simulink model "vaja04"  (R2013a)
settings: Solver=ode45  StartTime=0.0  StopTime=400  MaxStep=0.01  RelTol=1e-3
undefined symbols (not defined in the file or in its folder): bar, histogram_hitrost, norma
libraries: simulink x39
settings Model: Creator=Studenti  LastModifiedBy=Studenti

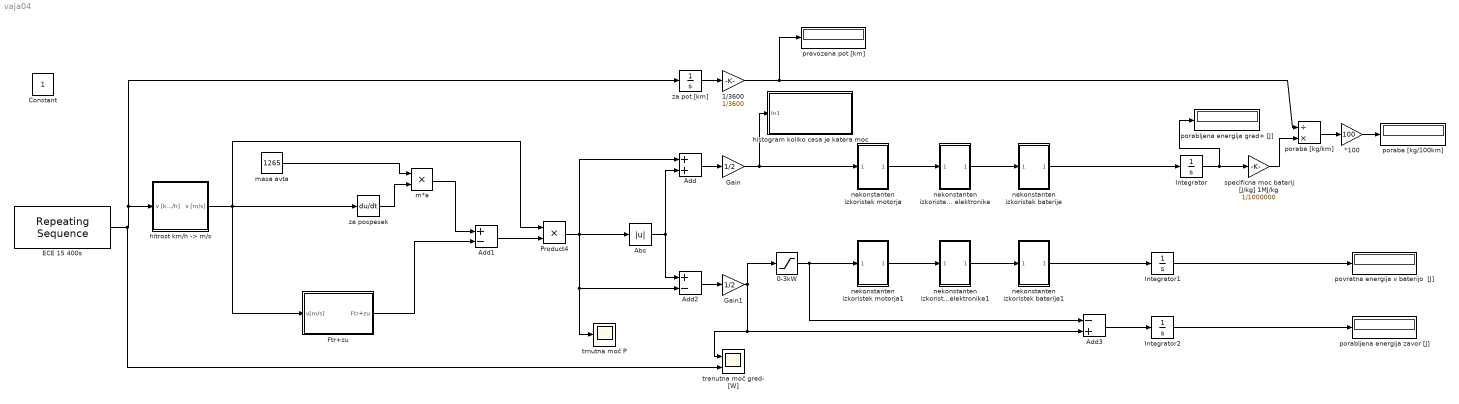
== system vaja04 ==
  *100 : Gain  Gain=100
  0-3kW : Saturate  UpperLimit=3000  LowerLimit=0
  1/3600 : Gain  Gain=1/3600
  Abs : Abs
  Add : Sum
  Add1 : Sum  Inputs=+-
  Add2 : Sum  Inputs=+-
  Add3 : Sum  Inputs=-+
  ECE 15 400s : simulink/Sources/Repeating Sequence  rep_seq_t=[0.0 11.3 15.0 23.2 28.2 48.9 60.8 85.2 95.9 117.2 142.8 154.8 162.9 176.0 188.0 200.0]  rep_seq_y=[0.0 0.0 5.0 5.0 0.0 0.0 32.0 32.0 0.0 0.0 50.0 50.0 35.0 35.0 0.0 0.0]
  Ftr+zu : Subsystem
  Gain : Gain  Gain=1/2
  Gain1 : Gain  Gain=1/2
  Integrator : Integrator
  Integrator1 : Integrator
  Integrator2 : Integrator
  Product4 : Product
  histogram koliko casa je katera moc : Subsystem  mask{obmocje=70000}
      mask prompts: obmocje "Vhodno območje"
  "hitrost km/h -> m/s" : Subsystem
  m*a : Product
  masa avta : Constant  Value=1265
  nekonstanten izkoristek baterije : Subsystem
  nekonstanten izkoristek baterije1 : Subsystem
  nekonstanten izkoristek elektronike : Subsystem
  nekonstanten izkoristek elektronike1 : Subsystem
  nekonstanten izkoristek motorja : Subsystem
  nekonstanten izkoristek motorja1 : Subsystem
  poraba [kg/100km] : Display
  poraba [kg/km] : Product  Inputs=/*
  porabljena energija gred+ [J] : Display
  porabljena energija zavor [J] : Display
  povratna energija v baterijo  [J] : Display
  prevozena pot [km] : Display
  specificna moc baterij [J/kg] 1MJ/kg : Gain  Gain=1/1000000
  trenutna moč gred- [W] : Scope  NumInputPorts=2
      settings: YMin=-5~-5  YMax=5~5
  trnutna moč P : Scope
  za pospesek : Derivative
  za pot [km] : Integrator
  Constant : Constant  IOType=siggen
  wires:
  ECE 15 400s/1 -> trenutna moč gred- [W]/2, za pot [km]/1, "hitrost km/h -> m/s"/1(v [km/h])
  za pospesek/1 -> m*a/2
  masa avta/1 -> m*a/1
  m*a/1 -> Add1/1
  Add1/1 -> Product4/2
  Product4/1 -> Add/1, Abs/1, trnutna moč P/1, Add2/2
  Ftr+zu/1(Ftr+zu) -> Add1/2
  Abs/1 -> Add2/1, Add/2
  specificna moc baterij [J/kg] 1MJ/kg/1 -> poraba [kg/km]/2
  poraba [kg/km]/1 -> *100/1
  *100/1 -> poraba [kg/100km]/1
  1/3600/1 -> prevozena pot [km]/1, poraba [kg/km]/1
  za pot [km]/1 -> 1/3600/1
  "hitrost km/h -> m/s"/1(v [m/s]) -> Product4/1, za pospesek/1, Ftr+zu/1(v[m/s])
  Integrator/1 -> porabljena energija gred+ [J]/1, specificna moc baterij [J/kg] 1MJ/kg/1
  Add/1 -> Gain/1
  Add2/1 -> Gain1/1
  Gain1/1 -> 0-3kW/1, Add3/2, trenutna moč gred- [W]/1
  Integrator1/1 -> povratna energija v baterijo  [J]/1
  0-3kW/1 -> nekonstanten izkoristek motorja1/1(In1), Add3/1
  Integrator2/1 -> porabljena energija zavor [J]/1
  Add3/1 -> Integrator2/1
  Gain/1 -> histogram koliko casa je katera moc/1(In1), nekonstanten izkoristek motorja/1(In1)
  nekonstanten izkoristek motorja/1(Out1) -> nekonstanten izkoristek elektronike/1(In1)
  nekonstanten izkoristek elektronike/1(Out1) -> nekonstanten izkoristek baterije/1(In1)
  nekonstanten izkoristek baterije/1(Out1) -> Integrator/1
  nekonstanten izkoristek motorja1/1(Out1) -> nekonstanten izkoristek elektronike1/1(In1)
  nekonstanten izkoristek elektronike1/1(Out1) -> nekonstanten izkoristek baterije1/1(In1)
  nekonstanten izkoristek baterije1/1(Out1) -> Integrator1/1

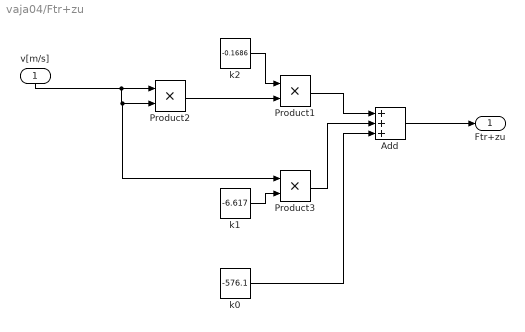
== system vaja04/Ftr+zu ==
  v[m/s] : Inport
  Add : Sum  Inputs=+++
  Product1 : Product
  Product2 : Product
  Product3 : Product
  k0 : Constant  Value=-576.1
  k1 : Constant  Value=-6.617
  k2 : Constant  Value=-0.1686
  Ftr+zu : Outport
  wires:
  k0/1 -> Add/3
  Product3/1 -> Add/2
  k2/1 -> Product1/1
  Product2/1 -> Product1/2
  Product1/1 -> Add/1
  Add/1 -> Ftr+zu/1
  k1/1 -> Product3/2
  v[m/s]/1 -> Product3/1, Product2/2, Product2/1

== system vaja04/histogram koliko casa je katera moc ==
  In1 : Inport
  Constant : Constant  Value=obmocje
  Divide : Product  Inputs=*/
  histogram : Subsystem  StopFcn=bar((0.025:0.05:0.975)*norma,histogram_hitrost)
  wires:
  Constant/1 -> Divide/2, histogram/2(norma)
  In1/1 -> Divide/1
  Divide/1 -> histogram/1(vhod)

== system vaja04/hitrost km//h -> m//s ==
  v [km/h] : Inport
  Product5 : Product
  "m/s " : Constant  Value=1/3.6
  v [m/s] : Outport
  wires:
  Product5/1 -> v [m/s]/1
  "m/s "/1 -> Product5/1
  v [km/h]/1 -> Product5/2

== system vaja04/nekonstanten izkoristek baterije ==
  In1 : Inport
  1-D Lookup Table : Lookup_n-D  NumberOfTableDimensions=1  BreakpointsForDimension1=[0 1]  Table=[0.99 0.93]  RndMeth=Simplest  InputSameDT=on
  1/70000 za normiranje moci : Gain  Gain=1/70000
  Divide : Product  Inputs=*/
  Out1 : Outport
  wires:
  In1/1 -> 1/70000 za normiranje moci/1, Divide/1
  1-D Lookup Table/1 -> Divide/2
  1/70000 za normiranje moci/1 -> 1-D Lookup Table/1
  Divide/1 -> Out1/1

== system vaja04/nekonstanten izkoristek baterije1 ==
  In1 : Inport
  1-D Lookup Table : Lookup_n-D  NumberOfTableDimensions=1  BreakpointsForDimension1=[0 1]  Table=[0.99 0.93]  RndMeth=Simplest  InputSameDT=on
  1/70000 za normiranje moci : Gain  Gain=1/70000
  Product : Product
  Out1 : Outport
  wires:
  In1/1 -> Product/1, 1/70000 za normiranje moci/1
  1-D Lookup Table/1 -> Product/2
  1/70000 za normiranje moci/1 -> 1-D Lookup Table/1
  Product/1 -> Out1/1

== system vaja04/nekonstanten izkoristek elektronike ==
  In1 : Inport
  1-D Lookup Table : Lookup_n-D  NumberOfTableDimensions=1  BreakpointsForDimension1=[0 0.02 0.5 1]  Table=[0.001 0.9 0.95 0.9]  RndMeth=Simplest  InputSameDT=on
  1/70000W za normiranje moci : Gain  Gain=1/70000
  Divide : Product  Inputs=*/
  Out1 : Outport
  wires:
  In1/1 -> 1/70000W za normiranje moci/1, Divide/1
  1-D Lookup Table/1 -> Divide/2
  1/70000W za normiranje moci/1 -> 1-D Lookup Table/1
  Divide/1 -> Out1/1

== system vaja04/nekonstanten izkoristek elektronike1 ==
  In1 : Inport
  1-D Lookup Table : Lookup_n-D  NumberOfTableDimensions=1  BreakpointsForDimension1=[0 0.02 0.5 1]  Table=[0.001 0.9 0.95 0.9]  RndMeth=Simplest  InputSameDT=on
  1/70000W za normiranje moci : Gain  Gain=1/70000
  Product : Product
  Out1 : Outport
  wires:
  In1/1 -> Product/1, 1/70000W za normiranje moci/1
  1-D Lookup Table/1 -> Product/2
  1/70000W za normiranje moci/1 -> 1-D Lookup Table/1
  Product/1 -> Out1/1

== system vaja04/nekonstanten izkoristek motorja ==
  In1 : Inport
  1-D Lookup Table : Lookup_n-D  NumberOfTableDimensions=1  BreakpointsForDimension1=[0 0.05 1]  Table=[0.001 0.95 0.6]  RndMeth=Simplest  InputSameDT=on
  1/70000 za normiranje moci : Gain  Gain=1/70000
  Divide : Product  Inputs=*/
  Out1 : Outport
  wires:
  In1/1 -> 1/70000 za normiranje moci/1, Divide/1
  1-D Lookup Table/1 -> Divide/2
  1/70000 za normiranje moci/1 -> 1-D Lookup Table/1
  Divide/1 -> Out1/1

== system vaja04/nekonstanten izkoristek motorja1 ==
  In1 : Inport
  1-D Lookup Table : Lookup_n-D  NumberOfTableDimensions=1  BreakpointsForDimension1=[0 0.05 1]  Table=[0.001 0.95 0.6]  RndMeth=Simplest  InputSameDT=on
  1/70000 za normiranje moci : Gain  Gain=1/70000
  Product : Product
  Out1 : Outport
  wires:
  In1/1 -> Product/1, 1/70000 za normiranje moci/1
  1-D Lookup Table/1 -> Product/2
  1/70000 za normiranje moci/1 -> 1-D Lookup Table/1
  Product/1 -> Out1/1

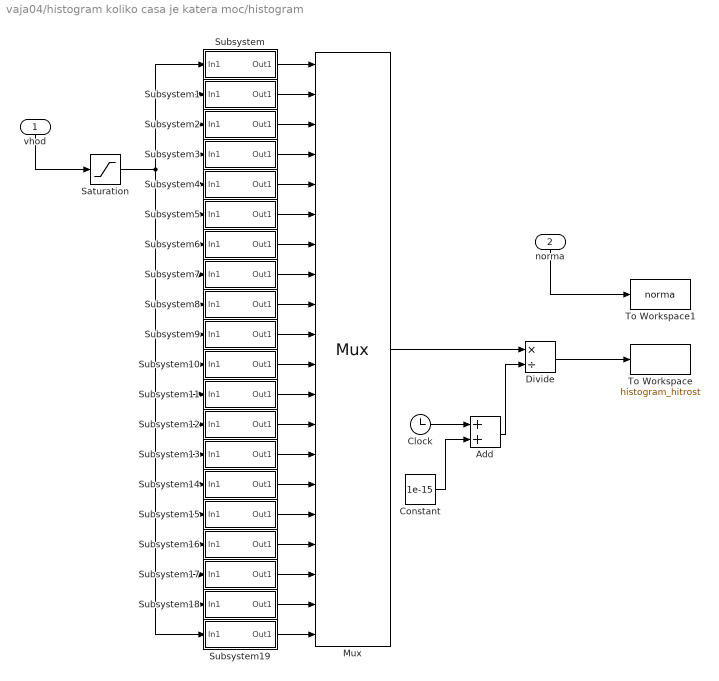
== system vaja04/histogram koliko casa je katera moc/histogram ==
  vhod : Inport
  norma : Inport  Port=2
  Add : Sum
  Clock : Clock
  Constant : Constant  Value=1e-15
  Divide : Product  Inputs=*/
  Mux : Mux  Inputs=20
  Saturation : Saturate  UpperLimit=1  LowerLimit=0
  Subsystem : Subsystem
  Subsystem1 : Subsystem
  Subsystem10 : Subsystem
  Subsystem11 : Subsystem
  Subsystem12 : Subsystem
  Subsystem13 : Subsystem
  Subsystem14 : Subsystem
  Subsystem15 : Subsystem
  Subsystem16 : Subsystem
  Subsystem17 : Subsystem
  Subsystem18 : Subsystem
  Subsystem19 : Subsystem
  Subsystem2 : Subsystem
  Subsystem3 : Subsystem
  Subsystem4 : Subsystem
  Subsystem5 : Subsystem
  Subsystem6 : Subsystem
  Subsystem7 : Subsystem
  Subsystem8 : Subsystem
  Subsystem9 : Subsystem
  To Workspace : ToWorkspace  VariableName=histogram_hitrost  SampleTime=-1
      settings: MaxDataPoints=1
  To Workspace1 : ToWorkspace  VariableName=norma  SampleTime=-1
      settings: MaxDataPoints=1
  wires:
  Divide/1 -> To Workspace/1
  vhod/1 -> Saturation/1
  Mux/1 -> Divide/1
  Clock/1 -> Add/1
  Add/1 -> Divide/2
  Constant/1 -> Add/2
  Subsystem/1(Out1) -> Mux/1
  Subsystem1/1(Out1) -> Mux/2
  Subsystem2/1(Out1) -> Mux/3
  Subsystem3/1(Out1) -> Mux/4
  Subsystem4/1(Out1) -> Mux/5
  Subsystem5/1(Out1) -> Mux/6
  Saturation/1 -> Subsystem/1(In1), Subsystem1/1(In1), Subsystem2/1(In1), Subsystem3/1(In1), Subsystem4/1(In1), Subsystem5/1(In1), Subsystem7/1(In1), Subsystem8/1(In1), Subsystem9/1(In1), Subsystem10/1(In1), Subsystem11/1(In1), Subsystem12/1(In1), Subsystem13/1(In1), Subsystem14/1(In1), Subsystem15/1(In1), Subsystem16/1(In1), Subsystem17/1(In1), Subsystem19/1(In1), Subsystem18/1(In1), Subsystem6/1(In1)
  Subsystem6/1(Out1) -> Mux/7
  Subsystem7/1(Out1) -> Mux/8
  Subsystem8/1(Out1) -> Mux/9
  Subsystem9/1(Out1) -> Mux/10
  Subsystem10/1(Out1) -> Mux/11
  Subsystem11/1(Out1) -> Mux/12
  Subsystem12/1(Out1) -> Mux/13
  Subsystem13/1(Out1) -> Mux/14
  Subsystem14/1(Out1) -> Mux/15
  Subsystem15/1(Out1) -> Mux/16
  Subsystem16/1(Out1) -> Mux/17
  Subsystem17/1(Out1) -> Mux/18
  Subsystem18/1(Out1) -> Mux/19
  Subsystem19/1(Out1) -> Mux/20
  norma/1 -> To Workspace1/1

== system vaja04/histogram koliko casa je katera moc/histogram/Subsystem ==
  In1 : Inport
  Compare To Constant1 : simulink/Logic and Bit Operations/Compare To Constant  relop=<  const=0.05  OutDataTypeStr=uint8  ZeroCross=off
  Data Type Conversion : DataTypeConversion  OutDataTypeStr=double
  Integrator : Integrator  ZeroCross=off
  Out1 : Outport
  wires:
  Data Type Conversion/1 -> Integrator/1
  Compare To Constant1/1 -> Data Type Conversion/1
  In1/1 -> Compare To Constant1/1
  Integrator/1 -> Out1/1

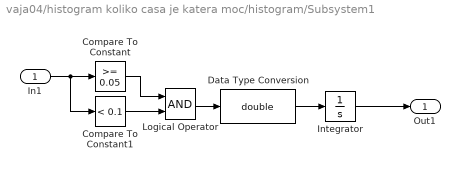
== system vaja04/histogram koliko casa je katera moc/histogram/Subsystem1 ==
  In1 : Inport
  Compare To Constant : simulink/Logic and Bit Operations/Compare To Constant  relop=>=  const=0.05  OutDataTypeStr=uint8  ZeroCross=off
  Compare To Constant1 : simulink/Logic and Bit Operations/Compare To Constant  relop=<  const=0.1  OutDataTypeStr=uint8  ZeroCross=off
  Data Type Conversion : DataTypeConversion  OutDataTypeStr=double
  Integrator : Integrator  ZeroCross=off
  Logical Operator : Logic  AllPortsSameDT=off  OutDataTypeStr=boolean
  Out1 : Outport
  wires:
  Data Type Conversion/1 -> Integrator/1
  Logical Operator/1 -> Data Type Conversion/1
  Compare To Constant/1 -> Logical Operator/1
  Compare To Constant1/1 -> Logical Operator/2
  In1/1 -> Compare To Constant/1, Compare To Constant1/1
  Integrator/1 -> Out1/1

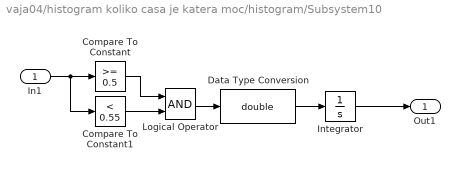
== system vaja04/histogram koliko casa je katera moc/histogram/Subsystem10 ==
  In1 : Inport
  Compare To Constant : simulink/Logic and Bit Operations/Compare To Constant  relop=>=  const=0.5  OutDataTypeStr=uint8  ZeroCross=off
  Compare To Constant1 : simulink/Logic and Bit Operations/Compare To Constant  relop=<  const=0.55  OutDataTypeStr=uint8  ZeroCross=off
  Data Type Conversion : DataTypeConversion  OutDataTypeStr=double
  Integrator : Integrator  ZeroCross=off
  Logical Operator : Logic  AllPortsSameDT=off  OutDataTypeStr=boolean
  Out1 : Outport
  wires:
  Data Type Conversion/1 -> Integrator/1
  Logical Operator/1 -> Data Type Conversion/1
  Compare To Constant/1 -> Logical Operator/1
  Compare To Constant1/1 -> Logical Operator/2
  In1/1 -> Compare To Constant/1, Compare To Constant1/1
  Integrator/1 -> Out1/1

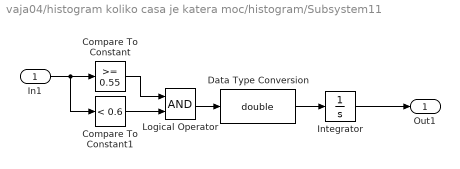
== system vaja04/histogram koliko casa je katera moc/histogram/Subsystem11 ==
  In1 : Inport
  Compare To Constant : simulink/Logic and Bit Operations/Compare To Constant  relop=>=  const=0.55  OutDataTypeStr=uint8  ZeroCross=off
  Compare To Constant1 : simulink/Logic and Bit Operations/Compare To Constant  relop=<  const=0.6  OutDataTypeStr=uint8  ZeroCross=off
  Data Type Conversion : DataTypeConversion  OutDataTypeStr=double
  Integrator : Integrator  ZeroCross=off
  Logical Operator : Logic  AllPortsSameDT=off  OutDataTypeStr=boolean
  Out1 : Outport
  wires:
  Data Type Conversion/1 -> Integrator/1
  Logical Operator/1 -> Data Type Conversion/1
  Compare To Constant/1 -> Logical Operator/1
  Compare To Constant1/1 -> Logical Operator/2
  In1/1 -> Compare To Constant/1, Compare To Constant1/1
  Integrator/1 -> Out1/1

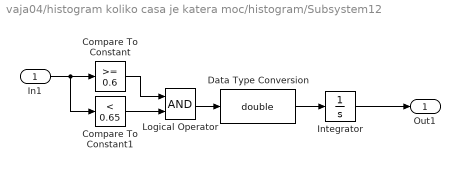
== system vaja04/histogram koliko casa je katera moc/histogram/Subsystem12 ==
  In1 : Inport
  Compare To Constant : simulink/Logic and Bit Operations/Compare To Constant  relop=>=  const=0.6  OutDataTypeStr=uint8  ZeroCross=off
  Compare To Constant1 : simulink/Logic and Bit Operations/Compare To Constant  relop=<  const=0.65  OutDataTypeStr=uint8  ZeroCross=off
  Data Type Conversion : DataTypeConversion  OutDataTypeStr=double
  Integrator : Integrator  ZeroCross=off
  Logical Operator : Logic  AllPortsSameDT=off  OutDataTypeStr=boolean
  Out1 : Outport
  wires:
  Data Type Conversion/1 -> Integrator/1
  Logical Operator/1 -> Data Type Conversion/1
  Compare To Constant/1 -> Logical Operator/1
  Compare To Constant1/1 -> Logical Operator/2
  In1/1 -> Compare To Constant/1, Compare To Constant1/1
  Integrator/1 -> Out1/1

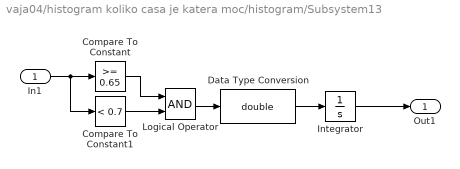
== system vaja04/histogram koliko casa je katera moc/histogram/Subsystem13 ==
  In1 : Inport
  Compare To Constant : simulink/Logic and Bit Operations/Compare To Constant  relop=>=  const=0.65  OutDataTypeStr=uint8  ZeroCross=off
  Compare To Constant1 : simulink/Logic and Bit Operations/Compare To Constant  relop=<  const=0.7  OutDataTypeStr=uint8  ZeroCross=off
  Data Type Conversion : DataTypeConversion  OutDataTypeStr=double
  Integrator : Integrator  ZeroCross=off
  Logical Operator : Logic  AllPortsSameDT=off  OutDataTypeStr=boolean
  Out1 : Outport
  wires:
  Data Type Conversion/1 -> Integrator/1
  Logical Operator/1 -> Data Type Conversion/1
  Compare To Constant/1 -> Logical Operator/1
  Compare To Constant1/1 -> Logical Operator/2
  In1/1 -> Compare To Constant/1, Compare To Constant1/1
  Integrator/1 -> Out1/1

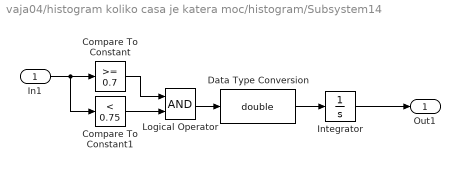
== system vaja04/histogram koliko casa je katera moc/histogram/Subsystem14 ==
  In1 : Inport
  Compare To Constant : simulink/Logic and Bit Operations/Compare To Constant  relop=>=  const=0.7  OutDataTypeStr=uint8  ZeroCross=off
  Compare To Constant1 : simulink/Logic and Bit Operations/Compare To Constant  relop=<  const=0.75  OutDataTypeStr=uint8  ZeroCross=off
  Data Type Conversion : DataTypeConversion  OutDataTypeStr=double
  Integrator : Integrator  ZeroCross=off
  Logical Operator : Logic  AllPortsSameDT=off  OutDataTypeStr=boolean
  Out1 : Outport
  wires:
  Data Type Conversion/1 -> Integrator/1
  Logical Operator/1 -> Data Type Conversion/1
  Compare To Constant/1 -> Logical Operator/1
  Compare To Constant1/1 -> Logical Operator/2
  In1/1 -> Compare To Constant/1, Compare To Constant1/1
  Integrator/1 -> Out1/1

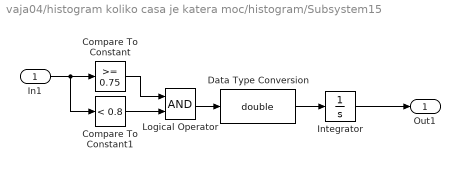
== system vaja04/histogram koliko casa je katera moc/histogram/Subsystem15 ==
  In1 : Inport
  Compare To Constant : simulink/Logic and Bit Operations/Compare To Constant  relop=>=  const=0.75  OutDataTypeStr=uint8  ZeroCross=off
  Compare To Constant1 : simulink/Logic and Bit Operations/Compare To Constant  relop=<  const=0.8  OutDataTypeStr=uint8  ZeroCross=off
  Data Type Conversion : DataTypeConversion  OutDataTypeStr=double
  Integrator : Integrator  ZeroCross=off
  Logical Operator : Logic  AllPortsSameDT=off  OutDataTypeStr=boolean
  Out1 : Outport
  wires:
  Data Type Conversion/1 -> Integrator/1
  Logical Operator/1 -> Data Type Conversion/1
  Compare To Constant/1 -> Logical Operator/1
  Compare To Constant1/1 -> Logical Operator/2
  In1/1 -> Compare To Constant/1, Compare To Constant1/1
  Integrator/1 -> Out1/1

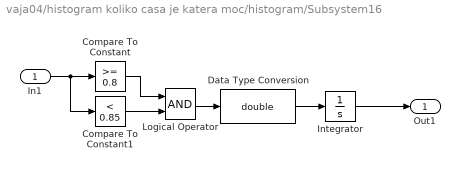
== system vaja04/histogram koliko casa je katera moc/histogram/Subsystem16 ==
  In1 : Inport
  Compare To Constant : simulink/Logic and Bit Operations/Compare To Constant  relop=>=  const=0.8  OutDataTypeStr=uint8  ZeroCross=off
  Compare To Constant1 : simulink/Logic and Bit Operations/Compare To Constant  relop=<  const=0.85  OutDataTypeStr=uint8  ZeroCross=off
  Data Type Conversion : DataTypeConversion  OutDataTypeStr=double
  Integrator : Integrator  ZeroCross=off
  Logical Operator : Logic  AllPortsSameDT=off  OutDataTypeStr=boolean
  Out1 : Outport
  wires:
  Data Type Conversion/1 -> Integrator/1
  Logical Operator/1 -> Data Type Conversion/1
  Compare To Constant/1 -> Logical Operator/1
  Compare To Constant1/1 -> Logical Operator/2
  In1/1 -> Compare To Constant/1, Compare To Constant1/1
  Integrator/1 -> Out1/1

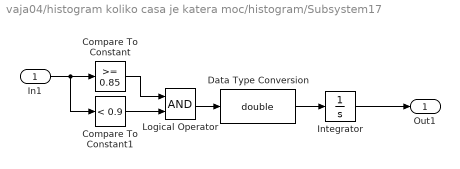
== system vaja04/histogram koliko casa je katera moc/histogram/Subsystem17 ==
  In1 : Inport
  Compare To Constant : simulink/Logic and Bit Operations/Compare To Constant  relop=>=  const=0.85  OutDataTypeStr=uint8  ZeroCross=off
  Compare To Constant1 : simulink/Logic and Bit Operations/Compare To Constant  relop=<  const=0.9  OutDataTypeStr=uint8  ZeroCross=off
  Data Type Conversion : DataTypeConversion  OutDataTypeStr=double
  Integrator : Integrator  ZeroCross=off
  Logical Operator : Logic  AllPortsSameDT=off  OutDataTypeStr=boolean
  Out1 : Outport
  wires:
  Data Type Conversion/1 -> Integrator/1
  Logical Operator/1 -> Data Type Conversion/1
  Compare To Constant/1 -> Logical Operator/1
  Compare To Constant1/1 -> Logical Operator/2
  In1/1 -> Compare To Constant/1, Compare To Constant1/1
  Integrator/1 -> Out1/1

== system vaja04/histogram koliko casa je katera moc/histogram/Subsystem18 ==
  In1 : Inport
  Compare To Constant : simulink/Logic and Bit Operations/Compare To Constant  relop=>=  const=0.9  OutDataTypeStr=uint8  ZeroCross=off
  Compare To Constant1 : simulink/Logic and Bit Operations/Compare To Constant  relop=<  const=0.95  OutDataTypeStr=uint8  ZeroCross=off
  Data Type Conversion : DataTypeConversion  OutDataTypeStr=double
  Integrator : Integrator  ZeroCross=off
  Logical Operator : Logic  AllPortsSameDT=off  OutDataTypeStr=boolean
  Out1 : Outport
  wires:
  Data Type Conversion/1 -> Integrator/1
  Logical Operator/1 -> Data Type Conversion/1
  Compare To Constant/1 -> Logical Operator/1
  Compare To Constant1/1 -> Logical Operator/2
  In1/1 -> Compare To Constant/1, Compare To Constant1/1
  Integrator/1 -> Out1/1

== system vaja04/histogram koliko casa je katera moc/histogram/Subsystem19 ==
  In1 : Inport
  Compare To Constant : simulink/Logic and Bit Operations/Compare To Constant  relop=>=  const=0.95  OutDataTypeStr=uint8  ZeroCross=off
  Data Type Conversion : DataTypeConversion  OutDataTypeStr=double
  Integrator : Integrator  ZeroCross=off
  Out1 : Outport
  wires:
  Data Type Conversion/1 -> Integrator/1
  Compare To Constant/1 -> Data Type Conversion/1
  In1/1 -> Compare To Constant/1
  Integrator/1 -> Out1/1

== system vaja04/histogram koliko casa je katera moc/histogram/Subsystem2 ==
  In1 : Inport
  Compare To Constant : simulink/Logic and Bit Operations/Compare To Constant  relop=>=  const=0.1  OutDataTypeStr=uint8  ZeroCross=off
  Compare To Constant1 : simulink/Logic and Bit Operations/Compare To Constant  relop=<  const=0.15  OutDataTypeStr=uint8  ZeroCross=off
  Data Type Conversion : DataTypeConversion  OutDataTypeStr=double
  Integrator : Integrator  ZeroCross=off
  Logical Operator : Logic  AllPortsSameDT=off  OutDataTypeStr=boolean
  Out1 : Outport
  wires:
  Data Type Conversion/1 -> Integrator/1
  Logical Operator/1 -> Data Type Conversion/1
  Compare To Constant/1 -> Logical Operator/1
  Compare To Constant1/1 -> Logical Operator/2
  In1/1 -> Compare To Constant/1, Compare To Constant1/1
  Integrator/1 -> Out1/1

== system vaja04/histogram koliko casa je katera moc/histogram/Subsystem3 ==
  In1 : Inport
  Compare To Constant : simulink/Logic and Bit Operations/Compare To Constant  relop=>=  const=0.15  OutDataTypeStr=uint8  ZeroCross=off
  Compare To Constant1 : simulink/Logic and Bit Operations/Compare To Constant  relop=<  const=0.2  OutDataTypeStr=uint8  ZeroCross=off
  Data Type Conversion : DataTypeConversion  OutDataTypeStr=double
  Integrator : Integrator  ZeroCross=off
  Logical Operator : Logic  AllPortsSameDT=off  OutDataTypeStr=boolean
  Out1 : Outport
  wires:
  Data Type Conversion/1 -> Integrator/1
  Logical Operator/1 -> Data Type Conversion/1
  Compare To Constant/1 -> Logical Operator/1
  Compare To Constant1/1 -> Logical Operator/2
  In1/1 -> Compare To Constant/1, Compare To Constant1/1
  Integrator/1 -> Out1/1

== system vaja04/histogram koliko casa je katera moc/histogram/Subsystem4 ==
  In1 : Inport
  Compare To Constant : simulink/Logic and Bit Operations/Compare To Constant  relop=>=  const=0.2  OutDataTypeStr=uint8  ZeroCross=off
  Compare To Constant1 : simulink/Logic and Bit Operations/Compare To Constant  relop=<  const=0.25  OutDataTypeStr=uint8  ZeroCross=off
  Data Type Conversion : DataTypeConversion  OutDataTypeStr=double
  Integrator : Integrator  ZeroCross=off
  Logical Operator : Logic  AllPortsSameDT=off  OutDataTypeStr=boolean
  Out1 : Outport
  wires:
  Data Type Conversion/1 -> Integrator/1
  Logical Operator/1 -> Data Type Conversion/1
  Compare To Constant/1 -> Logical Operator/1
  Compare To Constant1/1 -> Logical Operator/2
  In1/1 -> Compare To Constant/1, Compare To Constant1/1
  Integrator/1 -> Out1/1

== system vaja04/histogram koliko casa je katera moc/histogram/Subsystem5 ==
  In1 : Inport
  Compare To Constant : simulink/Logic and Bit Operations/Compare To Constant  relop=>=  const=0.25  OutDataTypeStr=uint8  ZeroCross=off
  Compare To Constant1 : simulink/Logic and Bit Operations/Compare To Constant  relop=<  const=0.3  OutDataTypeStr=uint8  ZeroCross=off
  Data Type Conversion : DataTypeConversion  OutDataTypeStr=double
  Integrator : Integrator  ZeroCross=off
  Logical Operator : Logic  AllPortsSameDT=off  OutDataTypeStr=boolean
  Out1 : Outport
  wires:
  Data Type Conversion/1 -> Integrator/1
  Logical Operator/1 -> Data Type Conversion/1
  Compare To Constant/1 -> Logical Operator/1
  Compare To Constant1/1 -> Logical Operator/2
  In1/1 -> Compare To Constant/1, Compare To Constant1/1
  Integrator/1 -> Out1/1

== system vaja04/histogram koliko casa je katera moc/histogram/Subsystem6 ==
  In1 : Inport
  Compare To Constant : simulink/Logic and Bit Operations/Compare To Constant  relop=>=  const=0.3  OutDataTypeStr=uint8  ZeroCross=off
  Compare To Constant1 : simulink/Logic and Bit Operations/Compare To Constant  relop=<  const=0.35  OutDataTypeStr=uint8  ZeroCross=off
  Data Type Conversion : DataTypeConversion  OutDataTypeStr=double
  Integrator : Integrator  ZeroCross=off
  Logical Operator : Logic  AllPortsSameDT=off  OutDataTypeStr=boolean
  Out1 : Outport
  wires:
  Data Type Conversion/1 -> Integrator/1
  Logical Operator/1 -> Data Type Conversion/1
  Compare To Constant/1 -> Logical Operator/1
  Compare To Constant1/1 -> Logical Operator/2
  In1/1 -> Compare To Constant/1, Compare To Constant1/1
  Integrator/1 -> Out1/1

== system vaja04/histogram koliko casa je katera moc/histogram/Subsystem7 ==
  In1 : Inport
  Compare To Constant : simulink/Logic and Bit Operations/Compare To Constant  relop=>=  const=0.35  OutDataTypeStr=uint8  ZeroCross=off
  Compare To Constant1 : simulink/Logic and Bit Operations/Compare To Constant  relop=<  const=0.4  OutDataTypeStr=uint8  ZeroCross=off
  Data Type Conversion : DataTypeConversion  OutDataTypeStr=double
  Integrator : Integrator  ZeroCross=off
  Logical Operator : Logic  AllPortsSameDT=off  OutDataTypeStr=boolean
  Out1 : Outport
  wires:
  Data Type Conversion/1 -> Integrator/1
  Logical Operator/1 -> Data Type Conversion/1
  Compare To Constant/1 -> Logical Operator/1
  Compare To Constant1/1 -> Logical Operator/2
  In1/1 -> Compare To Constant/1, Compare To Constant1/1
  Integrator/1 -> Out1/1

== system vaja04/histogram koliko casa je katera moc/histogram/Subsystem8 ==
  In1 : Inport
  Compare To Constant : simulink/Logic and Bit Operations/Compare To Constant  relop=>=  const=0.4  OutDataTypeStr=uint8  ZeroCross=off
  Compare To Constant1 : simulink/Logic and Bit Operations/Compare To Constant  relop=<  const=0.45  OutDataTypeStr=uint8  ZeroCross=off
  Data Type Conversion : DataTypeConversion  OutDataTypeStr=double
  Integrator : Integrator  ZeroCross=off
  Logical Operator : Logic  AllPortsSameDT=off  OutDataTypeStr=boolean
  Out1 : Outport
  wires:
  Data Type Conversion/1 -> Integrator/1
  Logical Operator/1 -> Data Type Conversion/1
  Compare To Constant/1 -> Logical Operator/1
  Compare To Constant1/1 -> Logical Operator/2
  In1/1 -> Compare To Constant/1, Compare To Constant1/1
  Integrator/1 -> Out1/1

== system vaja04/histogram koliko casa je katera moc/histogram/Subsystem9 ==
  In1 : Inport
  Compare To Constant : simulink/Logic and Bit Operations/Compare To Constant  relop=>=  const=0.45  OutDataTypeStr=uint8  ZeroCross=off
  Compare To Constant1 : simulink/Logic and Bit Operations/Compare To Constant  relop=<  const=0.5  OutDataTypeStr=uint8  ZeroCross=off
  Data Type Conversion : DataTypeConversion  OutDataTypeStr=double
  Integrator : Integrator  ZeroCross=off
  Logical Operator : Logic  AllPortsSameDT=off  OutDataTypeStr=boolean
  Out1 : Outport
  wires:
  Data Type Conversion/1 -> Integrator/1
  Logical Operator/1 -> Data Type Conversion/1
  Compare To Constant/1 -> Logical Operator/1
  Compare To Constant1/1 -> Logical Operator/2
  In1/1 -> Compare To Constant/1, Compare To Constant1/1
  Integrator/1 -> Out1/1
